simulink model "SIRV_V2_lm"  (R2023b)
settings: Solver=VariableStepAuto  StartTime=0.0  StopTime=200  RelTol=1e-3
settings Model: Creator=simon  LastModifiedBy=simon

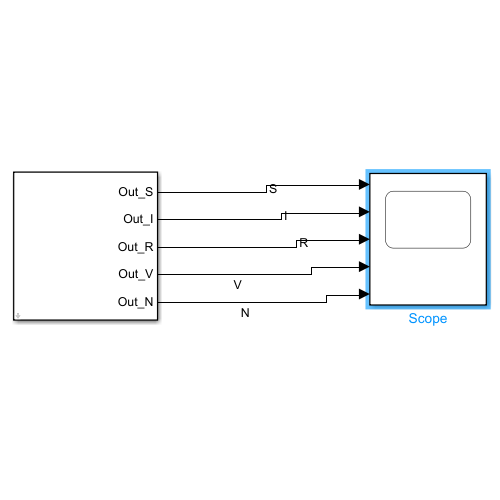
[thumbnail: Simulink's stored preview of the top-level diagram]
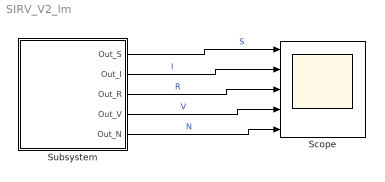
== system SIRV_V2_lm ==
  Scope : Scope  NumInputPorts=5
  Subsystem : Subsystem  mask{B=1e-4, p=0, Beta_=0.2, nu_=0, d=1e-4, gamma_=0, S_0=0.5, I_0=0.5*1e-4, R_0=0, V_0=0}
      mask prompts: B "Tasa de nacimientos (B)"; p "Proporcion de inmunzacion infantil (p)"; Beta_ "tasa de ... (β)"; nu_ "Tasa de vacunacion e inmunizacion (ν)"; d "Tasa de mortalidad natural (d)"; gamma_ "Tasa de recuperacion"; S_0 "Poblacion suceptible inicial"; I_0 "Poblacion infectada inicial"; R_0 "Poblacion recuperada inicial"; V_0 "Poblacion vacunada inicial"
  wires:
  Subsystem/3(Out_R) -> Scope/3  "R"
  Subsystem/4(Out_V) -> Scope/4  "V"
  Subsystem/1(Out_S) -> Scope/1  "S"
  Subsystem/2(Out_I) -> Scope/2  "I"
  Subsystem/5(Out_N) -> Scope/5  "N"

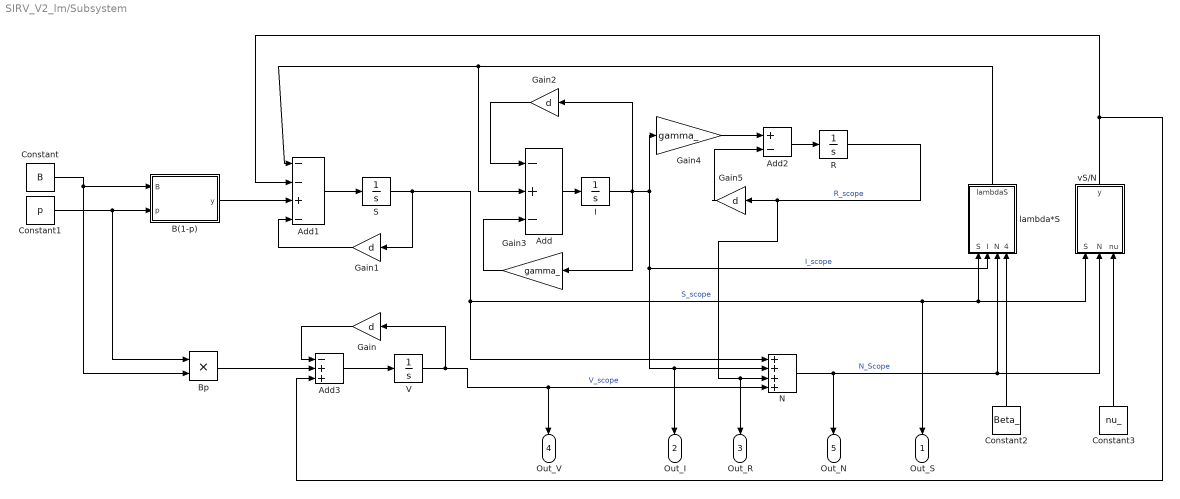
== system SIRV_V2_lm/Subsystem ==
  Add : Sum  Inputs=-+-
  Add1 : Sum  Inputs=--+-
  Add2 : Sum  Inputs=+-
  Add3 : Sum  Inputs=-++
  B(1-p) : MATLAB Function  TreatAsAtomicUnit=on
  Bp : Product
  Constant : Constant  Value=B
  Constant1 : Constant  Value=p
  Constant2 : Constant  Value=Beta_
  Constant3 : Constant  Value=nu_
  Gain{,1..2,5} (4 alike) : Gain  Gain=d
  Gain3 : Gain  Gain=gamma_
  Gain4 : Gain  Gain=gamma_
  I : Integrator  InitialCondition=I_0
  N : Sum  Inputs=++++
  R : Integrator  InitialCondition=R_0
  S : Integrator  InitialCondition=S_0
  V : Integrator  InitialCondition=V_0
  lambda*S : MATLAB Function  TreatAsAtomicUnit=on
  vS/N : MATLAB Function  TreatAsAtomicUnit=on
  Out_S : Outport
  Out_I : Outport  Port=2
  Out_R : Outport  Port=3
  Out_V : Outport  Port=4
  Out_N : Outport  Port=5
  wires:
  Gain/1 -> Add3/1
  Bp/1 -> Add3/2
  Constant2/1 -> lambda*S/4(beta)
  V/1 -> Out_V/1, N/4, Gain/1  "V_scope"
  Constant1/1 -> Bp/1, B(1-p)/2(p)
  Gain2/1 -> Add/1
  Gain5/1 -> Add2/2
  I/1 -> Gain4/1, N/2, Out_I/1, lambda*S/2(I), Gain3/1, Gain2/1  "I_scope"
  S/1 -> vS/N/1(S), lambda*S/1(S), Out_S/1, N/1, Gain1/1  "S_scope"
  N/1 -> vS/N/2(N), lambda*S/3(N), Out_N/1  "N_Scope"
  Gain3/1 -> Add/3
  R/1 -> N/3, Out_R/1, Gain5/1  "R_scope"
  B(1-p)/1(y) -> Add1/3
  Gain4/1 -> Add2/1
  Constant3/1 -> vS/N/3(nu)
  vS/N/1(y) -> Add3/3, Add1/2
  lambda*S/1(lambdaS) -> Add1/1, Add/2
  Constant/1 -> B(1-p)/1(B), Bp/2
  Add3/1 -> V/1
  Add2/1 -> R/1
  Add/1 -> I/1
  Add1/1 -> S/1
  Gain1/1 -> Add1/4

== matlab function SIRV_V2_lm/Subsystem/lambda*S ==
  data: S input; I input; N input; beta input; lambdaS output
function lambdaS = fcn(S,I,N,beta)

lambdaS = S*((beta*I)/N);

== matlab function SIRV_V2_lm/Subsystem/B(1-p) ==
  data: B input; y output; p input
function y = fcn(B,p)

y = B*(1-p);

== matlab function SIRV_V2_lm/Subsystem/vS//N ==
  data: S input; N input; nu input; y output
function y = fcn(S,N,nu)

y = (nu*S)/N;
